simulink model "MBSE_drone_project_stateflow"  (R2023a)
settings: Solver=FixedStepDiscrete  StartTime=0.0  StopTime=10.0  FixedStep=0.1  RelTol=1e-3  EnableMultiTasking=on
settings Model: Creator=Daniël  LastModifiedBy=Daniël
settings SolverCC: AlgebraicLoopSolver=TrustRegion  AutoInsertRateTranBlk=on
settings DataIOCC: LimitDataPoints=on
settings OptimizationCC: LifeSpan=inf
settings DebuggingCC: UnconnectedInputMsg=warning  UnconnectedOutputMsg=warning  UnconnectedLineMsg=warning  AllowSymbolicDim=off  SFUnexpectedBacktrackingDiag=warning  SFNoUnconditionalDefaultTransitionDiag=warning  SFExecutionAtInitializationDiag=none  ArithmeticOperatorsInVariantConditions=warning
settings ModelReferenceCC: EnableRefExpFcnMdlSchedulingChecks=on
settings SFSimCC: SimUseLocalCustomCode=off  CustomCodeUndefinedFunction=UseInterfaceOnly
settings RTWCC: RTWUseLocalCustomCode=off  DLArmComputeVersion=19.05
settings CodeAppCC: StateflowObjectComments=on
settings GRTTargetCC: TargetLangStandard=C89/C90 (ANSI)
settings ConfigComp: CovMetricSettings=dw  CovSaveCumulativeToWorkspaceVar=on  CovSaveSingleToWorkspaceVar=on  CovExternalEMLEnable=off  CovSFcnEnable=off

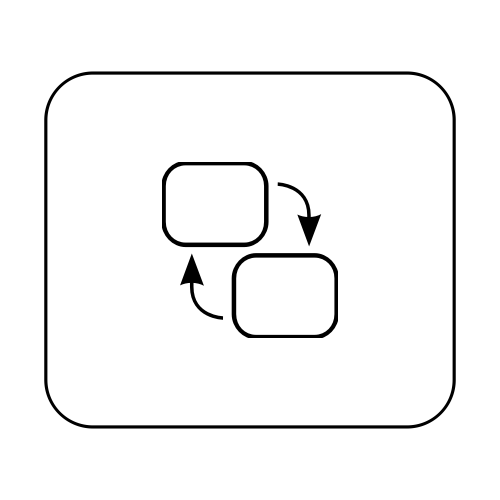
[thumbnail: Simulink's stored preview of the top-level diagram]
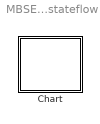
== system MBSE_drone_project_stateflow ==
  Chart : Stateflow chart  TreatAsAtomicUnit=on

== stateflow chart MBSE_drone_project_stateflow/Chart ==
  state HoverAtHome
    x=0
    y=0
    z=-1
    ld=0
    yaw=0
    loops=2
    loopsdone=0
    delay=2
  state Movefwd
    x=2
    y=0
    z=-1.3
    ld=0
  state Inspect
    x=2
    y=0
    z=-0.5
    ld=0
  state MoveUp
    x=2
    y=0
    z=-1.3
    ld=0
    yaw=3.1415
  state MoveToHome
    x=0
    y=0
    z=-1
    ld=0
  state PosHoldDrone
    z=-1
    yaw=0
    exit:loopsdone=loopdone+1
  state Land
    ld=1
  (default) -> HoverAtHome
  Movefwd -> Inspect : [(xes<=X+0.1)&&(xes<=x-0.1)&&(yes<=y+0.1)&&(yes<=y-0.1)&&(zes<z+0.1)&&(zes<=z-0.1)&&after(delay,sec)]
  Inspect -> MoveUp : [(xes<=X+0.1)&&(xes<=x-0.1)&&(yes<=y+0.1)&&(yes<=y-0.1)&&(zes<z+0.1)&&(zes<=z-0.1)&&after(delay,sec)]
  HoverAtHome -> Movefwd : [(xes<=X+0.1)&&(xes<=x-0.1)&&(yes<=y+0.1)&&(yes<=y-0.1)&&(zes<z+0.1)&&(zes<=z-0.1)&&after(delay,sec)]
  MoveUp -> MoveToHome : [(xes<=X+0.1)&&(xes<=x-0.1)&&(yes<=y+0.1)&&(yes<=y-0.1)&&(zes<z+0.1)&&(zes<=z-0.1)&&after(delay,sec)]
  MoveToHome -> PosHoldDrone : [(xes<=X+0.1)&&(xes<=x-0.1)&&(yes<=y+0.1)&&(yes<=y-0.1)&&(zes<z+0.1)&&(zes<=z-0.1)&&after(delay,sec)]
  (junction 19) -> Movefwd [order 2] : [loopsdone<=loops]
  PosHoldDrone -> (junction 19) : [(xes<=X+0.1)&&(xes<=x-0.1)&&(yes<=y+0.1)&&(yes<=y-0.1)&&(zes<z+0.1)&&(zes<=z-0.1)&&after(delay,sec)]
  (junction 19) -> Land [order 1] : [loops==loopsdone]
